simulink model "lqi_design_2019"  (R2021a)
settings: Solver=ode45  StartTime=0.0  StopTime=Tmax  RelTol=1e-6  EnableMultiTasking=on
values from neighbouring files (symbols this model uses):
  Ki = Kfull(:,1:3)    [lqe_system.m]    (also in lqigain.m)
  Ks = Kfull(:,4:15)    [lqe_system.m]    (also in lqigain.m)
undefined symbols (not defined in the file or in its folder): DiscIntNeverNeededParam, x0_quadcopter
settings Model: Creator=Mauricio  LastModifiedBy=martijndebeuf
settings SolverCC: AlgebraicLoopSolver=TrustRegion
settings DataIOCC: LimitDataPoints=on  SaveFormat=Array  ReturnWorkspaceOutputs=off
settings OptimizationCC: ExpressionDepthLimit=2147483647  LifeSpan=inf
settings DebuggingCC: UnderspecifiedInitializationDetection=Classic  MergeDetectMultiDrivingBlocksExec=none  SolverPrmCheckMsg=warning  StateNameClashWarn=warning  SFUnexpectedBacktrackingDiag=warning  SFNoUnconditionalDefaultTransitionDiag=warning  SFExecutionAtInitializationDiag=none  SFMachineParentedDataDiag=warning  ArithmeticOperatorsInVariantConditions=warning
settings HardwareCC: ProdBitPerPointer=32  ProdBitPerSizeT=32  ProdBitPerPtrDiffT=32  ProdLargestAtomicFloat=None  ProdIntDivRoundTo=Undefined  ProdEndianess=Unspecified  ProdWordSize=32  ProdHWDeviceType=32-bit Generic
settings ModelReferenceCC: PropagateSignalLabelsOutOfModel=off
settings SFSimCC: SimUseLocalCustomCode=off  CustomCodeUndefinedFunction=UseInterfaceOnly
settings RTWCC: RTWUseLocalCustomCode=off
settings CodeAppCC: StateflowObjectComments=on
settings GRTTargetCC: TargetLangStandard=C89/C90 (ANSI)
settings ConfigComp: CovMetricSettings=dw  CovSaveCumulativeToWorkspaceVar=on  CovSaveSingleToWorkspaceVar=on  CovExternalEMLEnable=off

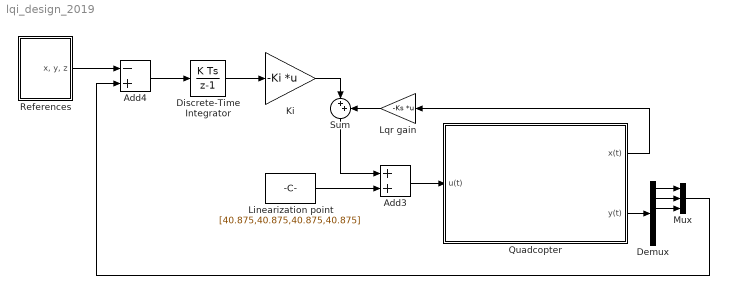
== system lqi_design_2019 ==
  Add3 : Sum
  Add4 : Sum  Inputs=-+
  Demux : Demux  Outputs=6
  Discrete-Time Integrator : DiscreteIntegrator  gainval=1  SampleTime=0.05  ICPrevOutput=DiscIntNeverNeededParam  ICPrevScaledInput=DiscIntNeverNeededParam
  "Ki " : Gain  Gain=-Ki  Multiplication=Matrix(K*u)
  Linearization point : Constant  Value=[40.875,40.875,40.875,40.875]  SampleTime=0.05
  "Lqr gain " : Gain  Gain=-Ks  Multiplication=Matrix(K*u)
  Mux : Mux  Inputs=3
  Quadcopter : Subsystem  mask(Quadcopter){x0=x0_quadcopter, sel_payload=0}
      mask prompts: x0 "Initial State - x0:"; sel_payload "Payload [kg]:"
      mask help:
      | u(t): Vector containing the squared voltages of the motors
      |
      | Oscar Mauricio Agudelo
      | (c) 2013
      mask init:
      | switch sel_payload
      |     case 1
      |        payload=0; 
      |     case 2
      |        payload=0.1; 
      |     otherwise
      |         payload=0;
      | end
      mask TypeOptions sel_payload: 0 | 0.1
      mask Display:
      | image(imread('icon_quad.png'));
      | port_label('input',1,'u(t)')
      | port_label('output',1,'x(t)')
      | port_label('output',2,'y(t)')
  References : Subsystem
  Sum : Sum  Inputs=|++
  wires:
  Add3/1 -> Quadcopter/1(u(t))
  Quadcopter/1(x(t)) -> "Lqr gain "/1
  Linearization point/1 -> Add3/2
  Discrete-Time Integrator/1 -> "Ki "/1
  Add4/1 -> Discrete-Time Integrator/1
  "Ki "/1 -> Sum/1
  Sum/1 -> Add3/1
  References/1("x, y, z") -> Add4/1
  Quadcopter/2(y(t)) -> Demux/1
  Mux/1 -> Add4/2
  Demux/1 -> Mux/1
  Demux/2 -> Mux/2
  Demux/3 -> Mux/3
  "Lqr gain "/1 -> Sum/2

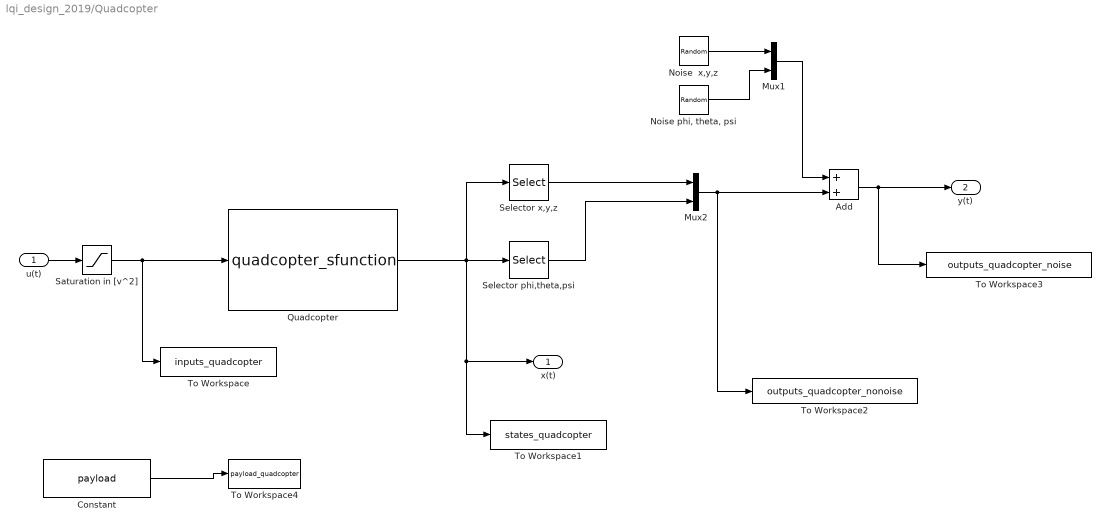
== system lqi_design_2019/Quadcopter ==
  u(t) : Inport
  Add : Sum
  Constant : Constant  Value=payload
  Mux1 : Mux  Inputs=2
  Mux2 : Mux  Inputs=2
  Noise  x,y,z : RandomNumber  Variance=[1 1 1]*(0.005)^2  SampleTime=0.05
  "Noise phi, theta, psi" : RandomNumber  Variance=[1 1 1]*(0.0087)^2  SampleTime=0.05
  Quadcopter : M-S-Function  FunctionName=quadcopter_sfunction  Parameters=x0, payload
  Saturation in [v^2] : Saturate  UpperLimit=100  LowerLimit=0
  Selector phi,theta,psi : Selector  IndexOptions=Index vector (dialog)  Indices=[7 8 9]  OutputSizes=1
  Selector x,y,z : Selector  IndexOptions=Index vector (dialog)  Indices=[1 2 3]  OutputSizes=1
  To Workspace : ToWorkspace  VariableName=inputs_quadcopter  SaveFormat=Structure With Time  SampleTime=-1
  To Workspace1 : ToWorkspace  VariableName=states_quadcopter  SaveFormat=Structure With Time  SampleTime=-1
  To Workspace2 : ToWorkspace  VariableName=outputs_quadcopter_nonoise  SaveFormat=Structure With Time  SampleTime=-1
  To Workspace3 : ToWorkspace  VariableName=outputs_quadcopter_noise  SaveFormat=Structure With Time  SampleTime=-1
  To Workspace4 : ToWorkspace  VariableName=payload_quadcopter  SampleTime=-1
  x(t) : Outport
  y(t) : Outport  Port=2
  wires:
  Saturation in [v^2]/1 -> Quadcopter/1, To Workspace/1
  u(t)/1 -> Saturation in [v^2]/1
  Mux2/1 -> To Workspace2/1, Add/2
  Selector phi,theta,psi/1 -> Mux2/2
  Selector x,y,z/1 -> Mux2/1
  Quadcopter/1 -> To Workspace1/1, x(t)/1, Selector x,y,z/1, Selector phi,theta,psi/1
  Add/1 -> To Workspace3/1, y(t)/1
  Noise  x,y,z/1 -> Mux1/1
  "Noise phi, theta, psi"/1 -> Mux1/2
  Mux1/1 -> Add/1
  Constant/1 -> To Workspace4/1

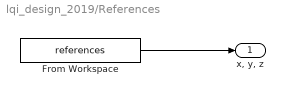
== system lqi_design_2019/References ==
  From Workspace : FromWorkspace  VariableName=references  SampleTime=0.1  Interpolate=off  OutputAfterFinalValue=Holding final value
  "x, y, z" : Outport
  wires:
  From Workspace/1 -> "x, y, z"/1
